simulink model "HIL_model"  (R2020b)
settings: Solver=VariableStepAuto  StartTime=0.0  StopTime=10.0  RelTol=1e-3
InitFcn:
  | Ts = 0.01;
  | IniT = 8;
  | FilterGain = 0.02;
libraries: arduinolib x2, arduinosensorlib x1, pid_lib x1
settings Model: Creator=Dallin  LastModifiedBy=Dallin

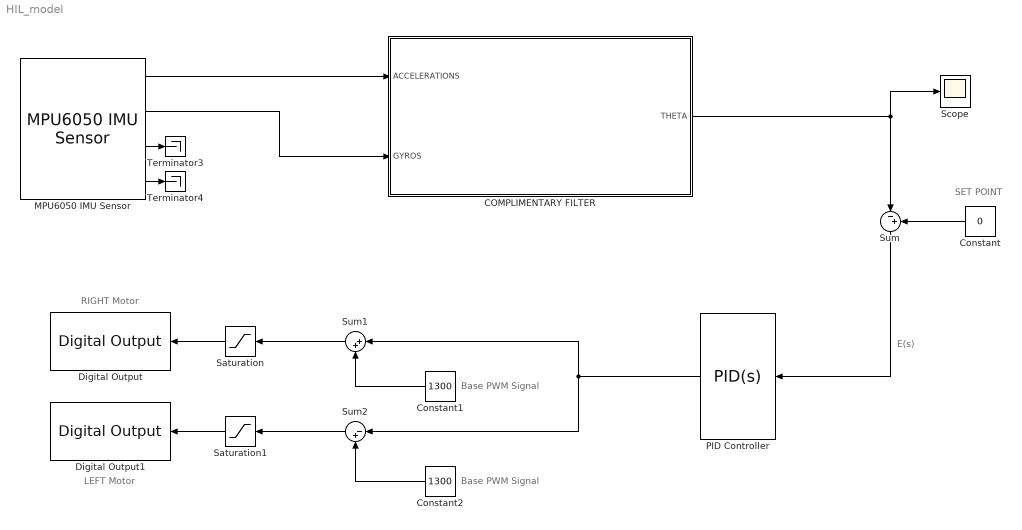
== system HIL_model ==
  note: E(s)
  note: LEFT Motor
  note: RIGHT Motor
  note: Base PWM Signal
  note: SET POINT
  note: Base PWM Signal
  COMPLIMENTARY FILTER : Subsystem
  Constant : Constant  Value=0
  Constant1 : Constant  Value=1300
  Constant2 : Constant  Value=1300
  Digital Output : arduinolib/Digital Output  pinNumber=3  Direction=output  blockPlatform=arduino
  Digital Output1 : arduinolib/Digital Output  pinNumber=5  Direction=output  blockPlatform=arduino
  MPU6050 IMU Sensor : arduinosensorlib/MPU6050 IMU Sensor  SlaveAddress=0x68  Accel=on  AngularRate=on  Temperature=on  Status=on  EulerAngles=off  Quat=off  AccelRange=2G  GyroRange=250 dps  DmpOdr=200 Hz  Dlpf=Accelerometer: 184Hz, Gyroscope: 188Hz  SampleTime=-1
      settings: SourceProductBaseCode=ARDUINO
  PID Controller : pid_lib/PID Controller  Controller=PID  Form=Parallel  TimeDomain=Continuous-time  UseExternalTs=off  SampleTime=-1  IntegratorMethod=Forward Euler  FilterMethod=Forward Euler  ControllerParametersSource=internal  P=1  I=1  D=0  UseFilter=on  N=100  TunerSelectOption=Transfer Function Based (PID Tuner App)  InitialConditionSource=internal  InitialConditionForIntegrator=0  InitialConditionForFilter=0  DifferentiatorICPrevScaledInput=0  ExternalReset=none  TrackingMode=off  Kt=1  LimitOutput=off  SatLimitsSource=internal  UpperSaturationLimit=inf  LowerSaturationLimit=-inf  LinearizeAsGain=on  AntiWindupMode=none  Kb=1  POutMin=[]  POutMax=[]  IOutMin=[]  IOutMax=[]  DOutMin=[]  DOutMax=[]  NOutMin=[]  NOutMax=[]  SumOutMin=[]  SumOutMax=[]  SaturationOutMin=[]  SaturationOutMax=[]  PParamMin=[]  PParamMax=[]  IParamMin=[]  IParamMax=[]  DParamMin=[]  DParamMax=[]  NParamMin=[]  NParamMax=[]  KbParamMin=[]  KbParamMax=[]  KtParamMin=[]  KtParamMax=[]  KbOutMin=[]  KbOutMax=[]  KtOutMin=[]  KtOutMax=[]  IntegratorOutMin=[]  IntegratorOutMax=[]  FilterOutMin=[]  FilterOutMax=[]  SumI1OutMin=[]  SumI1OutMax=[]  SumI2OutMin=[]  SumI2OutMax=[]  SumI3OutMin=[]  SumI3OutMax=[]  SumI4OutMin=[]  SumI4OutMax=[]  SumDOutMin=[]  SumDOutMax=[]  DifferentiatorOutMin=[]  DifferentiatorOutMax=[]  FilterDiffOutCoefMin=[]  FilterDiffOutCoefMax=[]  ReciprocalOutMin=[]  ReciprocalOutMax=[]  SumDenOutMin=[]  SumDenOutMax=[]  SumNumOutMin=[]  SumNumOutMax=[]  DivideOutMin=[]  DivideOutMax=[]  UdiffTsProdOutMin=[]  UdiffTsProdOutMax=[]  NTsProdOutMin=[]  NTsProdOutMax=[]  UintegralTsProdOutMin=[]  UintegralTsProdOutMax=[]  UngainTsProdOutMin=[]  UngainTsProdOutMax=[]  IntegratorContinuousStateAttributes=''  IntegratorStateMustResolveToSignalObject=off  IntegratorRTWStateStorageClass=Auto  FilterContinuousStateAttributes=''  FilterStateMustResolveToSignalObject=off  FilterRTWStateStorageClass=Auto  ParallelPVariant=InternalParameters  IdealPVariant=Disabled  IVariant=InternalParameters  DVariant=InternalParameters  IntegratorVariant=Continuous  SatVariant=Disabled  AWVariant=Passthrough  PCopyVariant=Disabled  TRVariant=Disabled  FdbkBlocksVariant=Forward  IdealPFdbkVariant=Disabled  SatFdbkVariant=Disabled  DerivativeFilterVariant=ContFilter  NVariant=InternalParameters  NCopyVariant=Disabled  FilterICVariant=InternalICsFilter  IntegratorICVariant=InternalICs  ExternalResetVariant=Disabled  TRSumVariant=Passthrough  SumFdbkVariant=Disabled  SumVariant=Sum_PID  TsampFilterVariant=InternalTs  TsampNgainVariant=Passthrough  TsampIntegralVariant=Passthrough  ExternalSaturationOutDataTypeStr=Inherit: Same as second input
  Saturation : Saturate  UpperLimit=2000  LowerLimit=1000
  Saturation1 : Saturate  UpperLimit=2000  LowerLimit=1000
  Scope : Scope
  Sum : Sum  Inputs=|-+
  Sum1 : Sum  Inputs=|++
  Sum2 : Sum  Inputs=|-+
  Terminator3 : Terminator
  Terminator4 : Terminator
  wires:
  MPU6050 IMU Sensor/3 -> Terminator3/1
  MPU6050 IMU Sensor/4 -> Terminator4/1
  Constant/1 -> Sum/2
  Sum/1 -> PID Controller/1
  Saturation/1 -> Digital Output/1
  Saturation1/1 -> Digital Output1/1
  Constant1/1 -> Sum1/2
  Constant2/1 -> Sum2/2
  Sum2/1 -> Saturation1/1
  Sum1/1 -> Saturation/1
  PID Controller/1 -> Sum2/1, Sum1/1
  COMPLIMENTARY FILTER/1(THETA) -> Sum/1, Scope/1
  MPU6050 IMU Sensor/1 -> COMPLIMENTARY FILTER/1(ACCELERATIONS)
  MPU6050 IMU Sensor/2 -> COMPLIMENTARY FILTER/2(GYROS)

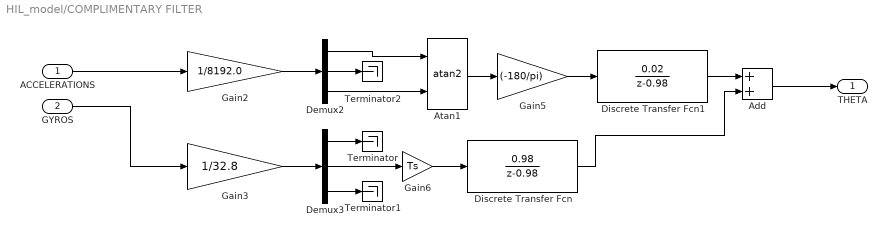
== system HIL_model/COMPLIMENTARY FILTER ==
  ACCELERATIONS : Inport
  GYROS : Inport  Port=2
  Add : Sum
  Atan1 : Trigonometry  Operator=atan2
  Demux2 : Demux  Outputs=3
  Demux3 : Demux  Outputs=3
  Discrete Transfer Fcn : DiscreteTransferFcn  Numerator=[0.98]  Denominator=[1 -0.98]
  Discrete Transfer Fcn1 : DiscreteTransferFcn  Numerator=[0.02]  Denominator=[1 -0.98]
  Gain2 : Gain  Gain=1/8192.0  OutDataTypeStr=double
  Gain3 : Gain  Gain=1/32.8  OutDataTypeStr=double
  Gain5 : Gain  Gain=(-180/pi)
  Gain6 : Gain  Gain=Ts
  Terminator : Terminator
  Terminator1 : Terminator
  Terminator2 : Terminator
  THETA : Outport
  wires:
  Demux2/1 -> Atan1/1
  Gain6/1 -> Discrete Transfer Fcn/1
  Gain2/1 -> Demux2/1
  Demux3/3 -> Terminator1/1
  Demux2/2 -> Terminator2/1
  Demux2/3 -> Atan1/2
  Discrete Transfer Fcn/1 -> Add/2
  Add/1 -> THETA/1
  Demux3/1 -> Terminator/1
  ACCELERATIONS/1 -> Gain2/1
  Discrete Transfer Fcn1/1 -> Add/1
  Gain5/1 -> Discrete Transfer Fcn1/1
  Atan1/1 -> Gain5/1
  Demux3/2 -> Gain6/1
  Gain3/1 -> Demux3/1
  GYROS/1 -> Gain3/1
